simulink model "CSEI"  (Simulink 7.3)
settings: Solver=ode4  StartTime=0.0  StopTime=Inf  FixedStep=0.1  RelTol=1e-3
values from neighbouring files (symbols this model uses):
  Ke = 100*diag([1.28 1.05 1.28 1.05 2.14])    [data.m]    (also in parameeters.m = diag([1.28 1.05 1.28 1.05 2.14]))
  Te = [1     0       1       0       0 ... (first row only)    [data.m]    (also in parameeters.m = [1 0 1 0 0; 0 1 0 1 1; ly1 -lx1 -ly2 -lx2 lx3])
undefined symbols (not defined in the file or in its folder): D, M
libraries: marine_gnc x6, simulink x5, simulink_extras x4
(part 1 of 2)
settings Model: Creator=hakonnod  LastModifiedBy=mcl  BufferReuse=off
settings DataIOCC: LimitDataPoints=off  SaveOutput=off  SignalLogging=off  SaveTime=off
settings OptimizationCC: BlockReduction=off  BooleanDataType=off  ConditionallyExecuteInputs=off  OptimizeBlockIOStorage=off  BufferReuse=off  ExpressionFolding=off  EnableMemcpy=off  LocalBlockOutputs=off  InitFltsAndDblsToZero=on  SimCompilerOptimization=On
settings ModelReferenceCC: UpdateModelReferenceTargets=Force
settings SFSimCC: SimBuildMode=sf_nonincremental_build
settings RTWCC: SystemTargetFile=nidll.tlc  TemplateMakefile=nidll_vc.tmf  Description=NI Real-Time Target for Release 2007b or later  ProcessScript=nidll_make_rtw_hook
settings STFCustomTargetCC: MatFileLogging=on  SystemTargetFile=nidll.tlc

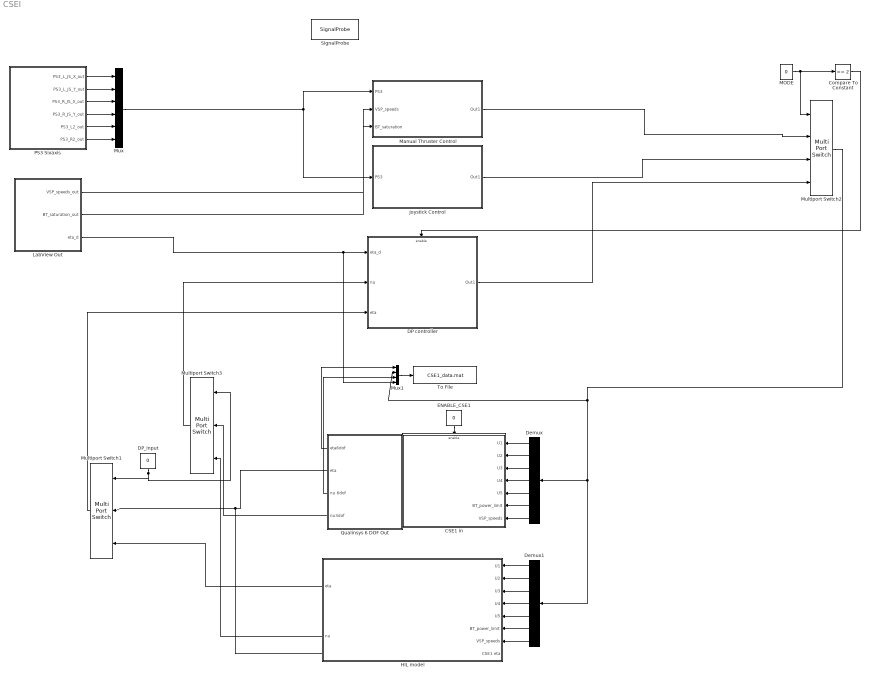
== system CSEI ==
  CSE1 in : Subsystem
  Compare To Constant : simulink/Logic and Bit Operations/Compare To Constant  SystemSampleTime=-1  relop===  const=2  LogicOutDataTypeMode=uint8
  DP controller : Subsystem
  DP_input : Constant  Value=0  OutDataType=fixdt(1, 16)  OutScaling=2^0
  Demux : Demux  Outputs=7
  Demux1 : Demux  Outputs=7
  ENABLE_CSE1 : Constant  Value=0  OutDataType=fixdt(1, 16)  OutScaling=2^0
  HIL model : Subsystem
  Joystick Control : Subsystem
  LabView Out : Subsystem
  MODE : Constant  Value=0  OutDataType=fixdt(1, 16)  OutScaling=2^0
  Manual Thruster Control : Subsystem
  Multiport Switch1 : MultiPortSwitch  Inputs=2  zeroidx=on  OutDataType=fixdt(1, 16)  OutScaling=2^0
  Multiport Switch2 : MultiPortSwitch  zeroidx=on  OutDataType=fixdt(1, 16)  OutScaling=2^0
  Multiport Switch3 : MultiPortSwitch  Inputs=2  zeroidx=on  OutDataType=fixdt(1, 16)  OutScaling=2^0
  Mux : Mux  Inputs=6
  Mux1 : Mux
  PS3 Sixaxis : Subsystem
  Qualinsys 6 DOF Out : Subsystem
  SignalProbe : S-Function  Description=Use this block with SIT.  FunctionName=SignalProbe  Parameters=1  EnableBusSupport=off
      settings: PreSaveFcn=NISIT_ModelVars;
      mask Description: The LabVIEW Simulation Interface Toolkit uses the SignalProbe block to probe the signals in the model. The SignalProbe block must be on the top level of the model hierarchy. You can have only one SignalProbe block per model file. Do not rename the SignalProbe block. Do not change the name of another model block to SignalProbe.
  To File : ToFile  Filename=CSE1_data.mat  MatrixName=cse1_data
  wires:
  PS3 Sixaxis/1(PS3_L_JS_X_out) -> Mux/1
  PS3 Sixaxis/2(PS3_L_JS_Y_out) -> Mux/2
  PS3 Sixaxis/3(PS3_R_JS_X_out) -> Mux/3
  PS3 Sixaxis/4(PS3_R_JS_Y_out) -> Mux/4
  PS3 Sixaxis/5(PS3_L2_out) -> Mux/5
  PS3 Sixaxis/6(PS3_R2_out) -> Mux/6
  Mux/1 -> Manual Thruster Control/1(PS3), Joystick Control/1(PS3)
  Manual Thruster Control/1(Out1) -> Multiport Switch2/2
  MODE/1 -> Multiport Switch2/1, Compare To Constant/1
  Multiport Switch2/1 -> Demux1/1, Demux/1, Mux1/2
  ENABLE_CSE1/1 -> CSE1 in/Enable
  DP controller/1(Out1) -> Multiport Switch2/4
  Compare To Constant/1 -> DP controller/Enable
  Joystick Control/1(Out1) -> Multiport Switch2/3
  Demux1/1 -> HIL model/1(U1)
  Demux1/2 -> HIL model/2(U2)
  Demux1/3 -> HIL model/3(U3)
  Demux1/4 -> HIL model/4(U4)
  Demux1/5 -> HIL model/5(U5)
  Demux1/6 -> HIL model/6(BT_power_limit)
  Demux1/7 -> HIL model/7(VSP_speeds)
  DP_input/1 -> Multiport Switch1/1, Multiport Switch3/1
  Qualinsys 6 DOF Out/2(eta) -> Multiport Switch1/2, HIL model/8(CSE1 eta)
  HIL model/1(eta) -> Multiport Switch1/3
  LabView Out/1(VSP_speeds_out) -> Manual Thruster Control/2(VSP_speeds)
  LabView Out/2(BT_saturation_out) -> Manual Thruster Control/3(BT_saturation)
  LabView Out/3(eta_d) -> DP controller/1(eta_d), Mux1/4
  HIL model/2(nu) -> Multiport Switch3/3
  Multiport Switch3/1 -> DP controller/2(nu)
  Mux1/1 -> To File/1
  Qualinsys 6 DOF Out/1(eta6dof) -> Mux1/1
  Demux/1 -> CSE1 in/1(U1)
  Demux/2 -> CSE1 in/2(U2)
  Demux/3 -> CSE1 in/3(U3)
  Demux/4 -> CSE1 in/4(U4)
  Demux/5 -> CSE1 in/5(U5)
  Demux/6 -> CSE1 in/6(BT_power_limit)
  Demux/7 -> CSE1 in/7(VSP_speeds)
  Qualinsys 6 DOF Out/4(nu3dof) -> Multiport Switch3/2
  Multiport Switch1/1 -> DP controller/3(eta)
  Qualinsys 6 DOF Out/3(nu 6dof) -> Mux1/3

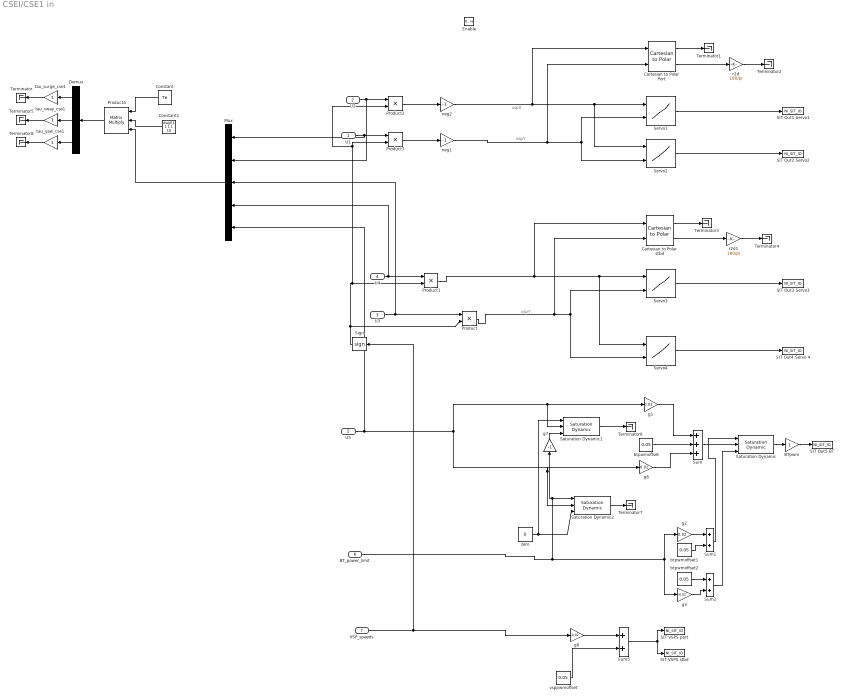
== system CSEI/CSE1 in ==
  note: vspX
  note: vspY
  note: vspY
  U1 : Inport  OutDataType=fixdt(1, 16)  OutScaling=2^0
  U2 : Inport  Port=2  OutDataType=fixdt(1, 16)  OutScaling=2^0
  U3 : Inport  Port=3  OutDataType=fixdt(1, 16)  OutScaling=2^0
  U4 : Inport  Port=4  OutDataType=fixdt(1, 16)  OutScaling=2^0
  U5 : Inport  Port=5  OutDataType=fixdt(1, 16)  OutScaling=2^0
  BT_power_limit : Inport  Port=6  OutDataType=fixdt(1, 16)  OutScaling=2^0
  VSP_speeds : Inport  Port=7  OutDataType=fixdt(1, 16)  OutScaling=2^0
  Enable : EnablePort
  BTpwm : Gain  ParameterDataType=fixdt(1, 16)  ParameterScaling=2^0  OutDataType=fixdt(1, 16)  OutScaling=2^0
  Cartesian to Polar Port : simulink_extras/Transformations/Cartesian to Polar  SystemSampleTime=-1
  Cartesian to Polar stbd : simulink_extras/Transformations/Cartesian to Polar  SystemSampleTime=-1
  Constant : Constant  Value=Te
  Constant1 : Constant  Value=diag([1 1 1 1 1])
  Demux : Demux  Outputs=3
  Mux : Mux  Inputs=5
  Product{,1..3} (4 alike) : Product  OutDataType=fixdt(1, 16)  OutScaling=2^0  RndMeth=Zero
  Product4 : Product  Inputs=3  Multiplication=Matrix(*)  RndMeth=Zero
  SIT Out1 Servo1 : S-Function  Priority=1  FunctionName=NI_SIT_IO  Parameters=width dtype portnum stime stype btype  EnableBusSupport=off  mask(SIT Outport){portnum=1, width=-1, stime=-1, dtype=auto, stype=auto, btype=0}
      mask prompts: portnum "Port number:"; width "Port dimensions (-1 for dynamically sized):"; stime "Sample time (-1 for inherited):"; dtype "Data type:"; stype "Signal type:"; btype "Block type:"
      mask help: Use this outport on any level of nested subsystems to allow the LabVIEW Simulation Interface Toolkit to map hardware to it.
      mask init:
      | NI_SIT_IO_init;
      settings: CopyFcn=NI_SIT_IO_callbacks(1);  DeleteFcn=NI_SIT_IO_callbacks(2);
      mask StyleString: edit,edit,edit,popup(auto|double|single|int8|uint8|int16|uint16|int32|uint32|boolean),popup(auto|real|complex),edit
      mask CallbackString: NI_SIT_IO_callbacks(3);|||NI_SIT_IO_callbacks(4);||
      mask TabNameString: Parameters,Parameters,Parameters,Parameters,Parameters,Parameters
      mask Display:
      | patch([-x x], [-y y], [.90980 .81960 .32156]);
      | plot([0 -x x 0], [rad -y y rad]);
      | fprintf('SIT%d', portnum);
  SIT Out2 Servo2 : S-Function  Priority=2  FunctionName=NI_SIT_IO  Parameters=width dtype portnum stime stype btype  EnableBusSupport=off  mask(SIT Outport){portnum=2, width=-1, stime=-1, dtype=auto, stype=auto, btype=0}
      mask prompts: portnum "Port number:"; width "Port dimensions (-1 for dynamically sized):"; stime "Sample time (-1 for inherited):"; dtype "Data type:"; stype "Signal type:"; btype "Block type:"
      mask help: Use this outport on any level of nested subsystems to allow the LabVIEW Simulation Interface Toolkit to map hardware to it.
      mask init:
      | NI_SIT_IO_init;
      settings: CopyFcn=NI_SIT_IO_callbacks(1);  DeleteFcn=NI_SIT_IO_callbacks(2);
      mask StyleString: edit,edit,edit,popup(auto|double|single|int8|uint8|int16|uint16|int32|uint32|boolean),popup(auto|real|complex),edit
      mask CallbackString: NI_SIT_IO_callbacks(3);|||NI_SIT_IO_callbacks(4);||
      mask TabNameString: Parameters,Parameters,Parameters,Parameters,Parameters,Parameters
      mask Display:
      | patch([-x x], [-y y], [.90980 .81960 .32156]);
      | plot([0 -x x 0], [rad -y y rad]);
      | fprintf('SIT%d', portnum);
  SIT Out3 Servo3 : S-Function  Priority=3  FunctionName=NI_SIT_IO  Parameters=width dtype portnum stime stype btype  EnableBusSupport=off  mask(SIT Outport){portnum=3, width=-1, stime=-1, dtype=auto, stype=auto, btype=0}
      mask prompts: portnum "Port number:"; width "Port dimensions (-1 for dynamically sized):"; stime "Sample time (-1 for inherited):"; dtype "Data type:"; stype "Signal type:"; btype "Block type:"
      mask help: Use this outport on any level of nested subsystems to allow the LabVIEW Simulation Interface Toolkit to map hardware to it.
      mask init:
      | NI_SIT_IO_init;
      settings: CopyFcn=NI_SIT_IO_callbacks(1);  DeleteFcn=NI_SIT_IO_callbacks(2);
      mask StyleString: edit,edit,edit,popup(auto|double|single|int8|uint8|int16|uint16|int32|uint32|boolean),popup(auto|real|complex),edit
      mask CallbackString: NI_SIT_IO_callbacks(3);|||NI_SIT_IO_callbacks(4);||
      mask TabNameString: Parameters,Parameters,Parameters,Parameters,Parameters,Parameters
      mask Display:
      | patch([-x x], [-y y], [.90980 .81960 .32156]);
      | plot([0 -x x 0], [rad -y y rad]);
      | fprintf('SIT%d', portnum);
  SIT Out4 Servo 4 : S-Function  Priority=4  FunctionName=NI_SIT_IO  Parameters=width dtype portnum stime stype btype  EnableBusSupport=off  mask(SIT Outport){portnum=4, width=-1, stime=-1, dtype=auto, stype=auto, btype=0}
      mask prompts: portnum "Port number:"; width "Port dimensions (-1 for dynamically sized):"; stime "Sample time (-1 for inherited):"; dtype "Data type:"; stype "Signal type:"; btype "Block type:"
      mask help: Use this outport on any level of nested subsystems to allow the LabVIEW Simulation Interface Toolkit to map hardware to it.
      mask init:
      | NI_SIT_IO_init;
      settings: CopyFcn=NI_SIT_IO_callbacks(1);  DeleteFcn=NI_SIT_IO_callbacks(2);
      mask StyleString: edit,edit,edit,popup(auto|double|single|int8|uint8|int16|uint16|int32|uint32|boolean),popup(auto|real|complex),edit
      mask CallbackString: NI_SIT_IO_callbacks(3);|||NI_SIT_IO_callbacks(4);||
      mask TabNameString: Parameters,Parameters,Parameters,Parameters,Parameters,Parameters
      mask Display:
      | patch([-x x], [-y y], [.90980 .81960 .32156]);
      | plot([0 -x x 0], [rad -y y rad]);
      | fprintf('SIT%d', portnum);
  SIT Out5 BT : S-Function  Priority=5  FunctionName=NI_SIT_IO  Parameters=width dtype portnum stime stype btype  EnableBusSupport=off  mask(SIT Outport){portnum=5, width=-1, stime=-1, dtype=auto, stype=auto, btype=0}
      mask prompts: portnum "Port number:"; width "Port dimensions (-1 for dynamically sized):"; stime "Sample time (-1 for inherited):"; dtype "Data type:"; stype "Signal type:"; btype "Block type:"
      mask help: Use this outport on any level of nested subsystems to allow the LabVIEW Simulation Interface Toolkit to map hardware to it.
      mask init:
      | NI_SIT_IO_init;
      settings: CopyFcn=NI_SIT_IO_callbacks(1);  DeleteFcn=NI_SIT_IO_callbacks(2);
      mask StyleString: edit,edit,edit,popup(auto|double|single|int8|uint8|int16|uint16|int32|uint32|boolean),popup(auto|real|complex),edit
      mask CallbackString: NI_SIT_IO_callbacks(3);|||NI_SIT_IO_callbacks(4);||
      mask TabNameString: Parameters,Parameters,Parameters,Parameters,Parameters,Parameters
      mask Display:
      | patch([-x x], [-y y], [.90980 .81960 .32156]);
      | plot([0 -x x 0], [rad -y y rad]);
      | fprintf('SIT%d', portnum);
  SIT VSPS port : S-Function  Priority=6  FunctionName=NI_SIT_IO  Parameters=width dtype portnum stime stype btype  EnableBusSupport=off  mask(SIT Outport){portnum=6, width=-1, stime=-1, dtype=auto, stype=auto, btype=0}
      mask prompts: portnum "Port number:"; width "Port dimensions (-1 for dynamically sized):"; stime "Sample time (-1 for inherited):"; dtype "Data type:"; stype "Signal type:"; btype "Block type:"
      mask help: Use this outport on any level of nested subsystems to allow the LabVIEW Simulation Interface Toolkit to map hardware to it.
      mask init:
      | NI_SIT_IO_init;
      settings: CopyFcn=NI_SIT_IO_callbacks(1);  DeleteFcn=NI_SIT_IO_callbacks(2);
      mask StyleString: edit,edit,edit,popup(auto|double|single|int8|uint8|int16|uint16|int32|uint32|boolean),popup(auto|real|complex),edit
      mask CallbackString: NI_SIT_IO_callbacks(3);|||NI_SIT_IO_callbacks(4);||
      mask TabNameString: Parameters,Parameters,Parameters,Parameters,Parameters,Parameters
      mask Display:
      | patch([-x x], [-y y], [.90980 .81960 .32156]);
      | plot([0 -x x 0], [rad -y y rad]);
      | fprintf('SIT%d', portnum);
  SIT VSPS stbd : S-Function  Priority=7  FunctionName=NI_SIT_IO  Parameters=width dtype portnum stime stype btype  EnableBusSupport=off  mask(SIT Outport){portnum=7, width=-1, stime=-1, dtype=auto, stype=auto, btype=0}
      mask prompts: portnum "Port number:"; width "Port dimensions (-1 for dynamically sized):"; stime "Sample time (-1 for inherited):"; dtype "Data type:"; stype "Signal type:"; btype "Block type:"
      mask help: Use this outport on any level of nested subsystems to allow the LabVIEW Simulation Interface Toolkit to map hardware to it.
      mask init:
      | NI_SIT_IO_init;
      settings: CopyFcn=NI_SIT_IO_callbacks(1);  DeleteFcn=NI_SIT_IO_callbacks(2);
      mask StyleString: edit,edit,edit,popup(auto|double|single|int8|uint8|int16|uint16|int32|uint32|boolean),popup(auto|real|complex),edit
      mask CallbackString: NI_SIT_IO_callbacks(3);|||NI_SIT_IO_callbacks(4);||
      mask TabNameString: Parameters,Parameters,Parameters,Parameters,Parameters,Parameters
      mask Display:
      | patch([-x x], [-y y], [.90980 .81960 .32156]);
      | plot([0 -x x 0], [rad -y y rad]);
      | fprintf('SIT%d', portnum);
  Saturation Dynamic : simulink/Discontinuities/Saturation Dynamic  SystemSampleTime=-1  OutMin=[]  OutMax=[]  OutDataTypeStr=Inherit: Same as second input  OutDataType=fixdt(1, 16)  OutScaling=2^-10  DoSatur=off
  Saturation Dynamic1 : simulink/Discontinuities/Saturation Dynamic  SystemSampleTime=-1  OutMin=[]  OutMax=[]  OutDataTypeStr=Inherit: Same as second input  OutDataType=fixdt(1, 16)  OutScaling=2^-10  DoSatur=off
  Saturation Dynamic2 : simulink/Discontinuities/Saturation Dynamic  SystemSampleTime=-1  OutMin=[]  OutMax=[]  OutDataTypeStr=Inherit: Same as second input  OutDataType=fixdt(1, 16)  OutScaling=2^-10  DoSatur=off
  Servo1 : Lookup2D  RowIndex=[-1,0,1]  ColumnIndex=[-1,0,1]  Table=reshape([0.06,0.0495363,0.043301,0.06,0.052446,0.043301,0.06,0.0541518,0.043301],3,3)  OutDataType=fixdt(1, 16)  OutScaling=2^0
  Servo2 : Lookup2D  RowIndex=[-1,0,1]  ColumnIndex=[-1,0,1]  Table=reshape([0.03860880,0.0386088,0.03860880,0.0459941,0.0477243,0.0500953,0.057,0.057,0.057],3,3)  OutDataType=fixdt(1, 16)  OutScaling=2^0
  Servo3 : Lookup2D  RowIndex=[-1,0,1]  ColumnIndex=[-1,0,1]  Table=reshape([0.0640809,0.0640809,0.0640809,0.0539629,0.0541315,0.0556492,0.0442664,0.0442664,0.0442664],3,3)  OutDataType=fixdt(1, 16)  OutScaling=2^0
  Servo4 : Lookup2D  RowIndex=[-1,0,1]  ColumnIndex=[-1,0,1]  Table=reshape([0.0602867,0.0470489,0.0403879,0.0602867,0.049747,0.0403879,0.0602867,0.0526138,0.0403879],3,3)  OutDataType=fixdt(1, 16)  OutScaling=2^0
  Sign : Signum
  Sum : Sum  Inputs=+++  OutDataType=fixdt(1, 16)  OutScaling=2^0
  Sum1 : Sum  OutDataType=fixdt(1, 16)  OutScaling=2^0
  Sum2 : Sum  OutDataType=fixdt(1, 16)  OutScaling=2^0
  Sum5 : Sum  OutDataType=fixdt(1, 16)  OutScaling=2^0
  Terminator{,1..8} (9 alike) : Terminator
  btpwmoffset : Constant  Value=0.05  OutDataType=fixdt(1, 16)  OutScaling=2^0
  btpwmoffset1 : Constant  Value=0.05  OutDataType=fixdt(1, 16)  OutScaling=2^0
  btpwmoffset2 : Constant  Value=0.05  OutDataType=fixdt(1, 16)  OutScaling=2^0
  g1 : Gain  Gain=0.02  ParameterDataType=fixdt(1, 16)  ParameterScaling=2^0  OutDataType=fixdt(1, 16)  OutScaling=2^0
  g2 : Gain  Gain=0.02  ParameterDataType=fixdt(1, 16)  ParameterScaling=2^0  OutDataType=fixdt(1, 16)  OutScaling=2^0
  g3 : Gain  Gain=-0.02  ParameterDataType=fixdt(1, 16)  ParameterScaling=2^0  OutDataType=fixdt(1, 16)  OutScaling=2^0
  g6 : Gain  Gain=0.02  ParameterDataType=fixdt(1, 16)  ParameterScaling=2^0  OutDataType=fixdt(1, 16)  OutScaling=2^0
  g7 : Gain  Gain=-1  ParameterDataType=fixdt(1, 16)  ParameterScaling=2^0  OutDataType=fixdt(1, 16)  OutScaling=2^0
  g8 : Gain  Gain=-0.02  ParameterDataType=fixdt(1, 16)  ParameterScaling=2^0  OutDataType=fixdt(1, 16)  OutScaling=2^0
  neg1 : Gain  Gain=-1  ParameterDataType=fixdt(1, 16)  ParameterScaling=2^0  OutDataType=fixdt(1, 16)  OutScaling=2^0
  neg2 : Gain  Gain=-1  ParameterDataType=fixdt(1, 16)  ParameterScaling=2^0  OutDataType=fixdt(1, 16)  OutScaling=2^0
  r2d : Gain  Gain=180/pi  ParameterDataType=fixdt(1, 16)  ParameterScaling=2^0  OutDataType=fixdt(1, 16)  OutScaling=2^0
  r2d1 : Gain  Gain=180/pi  ParameterDataType=fixdt(1, 16)  ParameterScaling=2^0  OutDataType=fixdt(1, 16)  OutScaling=2^0
  tau_surge_cse1 : Gain  ParameterDataType=fixdt(1, 16)  ParameterScaling=2^0  OutDataType=fixdt(1, 16)  OutScaling=2^0
  tau_sway_cse1 : Gain  ParameterDataType=fixdt(1, 16)  ParameterScaling=2^0  OutDataType=fixdt(1, 16)  OutScaling=2^0
  tau_yaw_cse1 : Gain  ParameterDataType=fixdt(1, 16)  ParameterScaling=2^0  OutDataType=fixdt(1, 16)  OutScaling=2^0
  vsppwmoffset : Constant  Value=0.05  OutDataType=fixdt(1, 16)  OutScaling=2^0
  zero : Constant  Value=0  OutDataType=fixdt(1, 16)  OutScaling=2^0
  wires:
  Servo1/1 -> SIT Out1 Servo1/1
  Servo2/1 -> SIT Out2 Servo2/1
  Cartesian to Polar Port/1 -> Terminator1/1
  Cartesian to Polar Port/2 -> r2d/1
  r2d/1 -> Terminator2/1
  neg2/1 -> Servo1/1, Servo2/1, Cartesian to Polar Port/1
  neg1/1 -> Servo1/2, Servo2/2, Cartesian to Polar Port/2
  Servo3/1 -> SIT Out3 Servo3/1
  Servo4/1 -> SIT Out4 Servo 4/1
  Cartesian to Polar stbd/1 -> Terminator3/1
  Cartesian to Polar stbd/2 -> r2d1/1
  r2d1/1 -> Terminator4/1
  BTpwm/1 -> SIT Out5 BT/1
  Sum/1 -> Saturation Dynamic/2
  Saturation Dynamic/1 -> BTpwm/1
  BT_power_limit/1 -> g2/1, g3/1, Saturation Dynamic2/1, g7/1
  btpwmoffset1/1 -> Sum1/2
  g2/1 -> Sum1/1
  Sum1/1 -> Saturation Dynamic/1
  g3/1 -> Sum2/2
  btpwmoffset2/1 -> Sum2/1
  Sum2/1 -> Saturation Dynamic/3
  Saturation Dynamic1/1 -> Terminator6/1
  Saturation Dynamic2/1 -> Terminator7/1
  zero/1 -> Saturation Dynamic2/3, Saturation Dynamic1/1
  g1/1 -> Sum/1
  btpwmoffset/1 -> Sum/2
  g6/1 -> Sum/3
  g7/1 -> Saturation Dynamic1/3
  U5/1 -> Saturation Dynamic1/2, g1/1, Saturation Dynamic2/2, g6/1, Mux/5
  vsppwmoffset/1 -> Sum5/2
  Sum5/1 -> SIT VSPS port/1, SIT VSPS stbd/1
  g8/1 -> Sum5/1
  VSP_speeds/1 -> g8/1, Sign/1
  U3/1 -> Product/1, Mux/3
  Product/1 -> Servo3/2, Servo4/2, Cartesian to Polar stbd/2
  Sign/1 -> Product/2, Product1/2, Product3/2, Product2/2
  U4/1 -> Product1/1, Mux/4
  Product1/1 -> Servo3/1, Servo4/1, Cartesian to Polar stbd/1
  U2/1 -> Product2/1, Mux/2
  U1/1 -> Product3/1, Mux/1
  Product2/1 -> neg2/1
  Product3/1 -> neg1/1
  Constant1/1 -> Product4/2
  Constant/1 -> Product4/1
  Demux/1 -> tau_surge_cse1/1
  Demux/2 -> tau_sway_cse1/1
  Demux/3 -> tau_yaw_cse1/1
  Product4/1 -> Demux/1
  tau_surge_cse1/1 -> Terminator/1
  tau_sway_cse1/1 -> Terminator5/1
  tau_yaw_cse1/1 -> Terminator8/1
  Mux/1 -> Product4/3

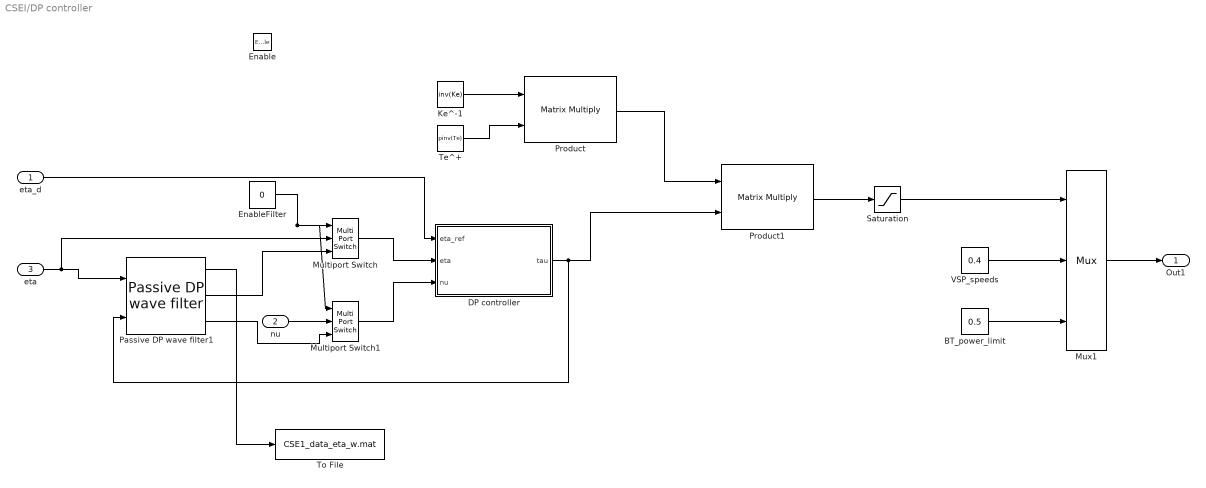
== system CSEI/DP controller ==
  eta_d : Inport  OutDataType=fixdt(1, 16)  OutScaling=2^0
  nu : Inport  Port=2  OutDataType=fixdt(1, 16)  OutScaling=2^0
  eta : Inport  Port=3  OutDataType=fixdt(1, 16)  OutScaling=2^0
  Enable : EnablePort  StatesWhenEnabling=reset
  BT_power_limit : Constant  Value=0.5  OutDataType=fixdt(1, 16)  OutScaling=2^0
  DP controller : Subsystem  mask(Nonlinear DP Controller){Kp=(0.1)^2*[25.8000 0  0;  0  33.8000  1.0115;  0  1.0115  2.7600 ], Kd=2*0.8*0.1*[25.8000 0  0;  0  33.8000  1.0115;  0  1.0115  2.7600 ], Ki=(0.1^3/10)*[25.8000 0  0;  0  33.8000  1.0115;  0  1.0115  2.7600 ]}
      mask prompts: Kp "Proportional Gain Matrix: Kp"; Kd "Derivative Gain Matrix: Kd"; Ki "Integral Gain Matrix: Ki"
      mask help: Nonlinear PID controller for Set-Point Reulation in Surge, Sway and Yaw
      mask Help:
      | The nonlinear  PID controller uses the rotation matrix in yaw for proper scaling of the surge, sway and yaw gains as a function of the yaw angle.
      | INPUTS: (1) eta_ref, (2) eta, (3) nu. OUPUTS: (1) tau.
      mask Display: disp('Nonlinear PID\n set-point controller')
  EnableFilter : Constant  Value=0  OutDataType=fixdt(1, 16)  OutScaling=2^0
  Ke^-1 : Constant  Value=inv(Ke)  OutDataType=fixdt(1, 16)  OutScaling=2^0
  Multiport Switch : MultiPortSwitch  Inputs=2  zeroidx=on  OutDataType=fixdt(1, 16)  OutScaling=2^0
  Multiport Switch1 : MultiPortSwitch  Inputs=2  zeroidx=on  OutDataType=fixdt(1, 16)  OutScaling=2^0
  Mux1 : Mux  Inputs=3
  Passive DP wave filter1 : marine_gnc/Navigation/Observers/Passive DP wave filter  SystemSampleTime=-1  lambda=0.1*diag([1 1 1])  w_o=diag([0.8 0.8 0.8])  K4=0.1*diag([1 1 0.1])  K3=0.1*diag([1 1 0.1])  w_c=1.3*diag([0.8 0.8 0.8])  T_b=diag([100 100 100])  M="[ 25.8000   0    0;   0   33.8000   1.0115; 0   1.0115    2.7600 ]"  D="[2 0  0;  0 7 0.1; 0 0.1 0.5]"
  Product : Product  Multiplication=Matrix(*)  OutDataType=fixdt(1, 16)  OutScaling=2^0  RndMeth=Zero
  Product1 : Product  Multiplication=Matrix(*)  OutDataType=fixdt(1, 16)  OutScaling=2^0  RndMeth=Zero
  Saturation : Saturate  UpperLimit=1.0  LowerLimit=-1.0  OutDataType=fixdt(1, 16)  OutScaling=2^0
  Te^+ : Constant  Value=pinv(Te)  OutDataType=fixdt(1, 16)  OutScaling=2^0
  To File : ToFile  Filename=CSE1_data_eta_w.mat  MatrixName=cse1_data
  VSP_speeds : Constant  Value=0.4  OutDataType=fixdt(1, 16)  OutScaling=2^0
  Out1 : Outport  OutDataType=fixdt(1, 16)  OutScaling=2^0
  wires:
  Product/1 -> Product1/1
  DP controller/1(tau) -> Product1/2, Passive DP wave filter1/2
  Ke^-1/1 -> Product/1
  Te^+/1 -> Product/2
  Mux1/1 -> Out1/1
  VSP_speeds/1 -> Mux1/2
  BT_power_limit/1 -> Mux1/3
  eta_d/1 -> DP controller/1(eta_ref)
  eta/1 -> Passive DP wave filter1/1, Multiport Switch/2
  nu/1 -> Multiport Switch1/2
  Multiport Switch/1 -> DP controller/2(eta)
  Multiport Switch1/1 -> DP controller/3(nu)
  Passive DP wave filter1/2 -> Multiport Switch/3
  Passive DP wave filter1/3 -> Multiport Switch1/3
  EnableFilter/1 -> Multiport Switch/1, Multiport Switch1/1
  Product1/1 -> Saturation/1
  Saturation/1 -> Mux1/1
  Passive DP wave filter1/1 -> To File/1

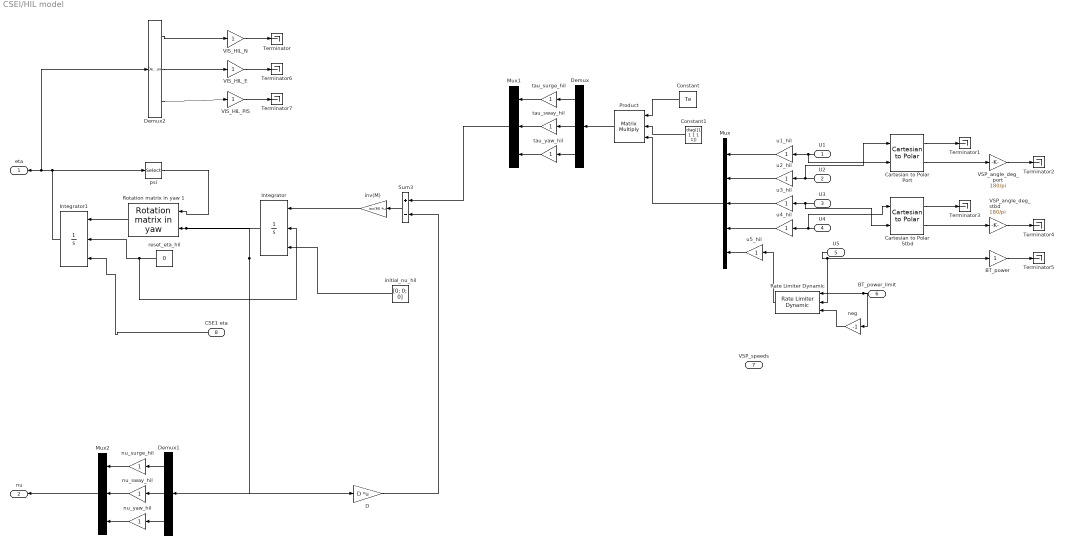
== system CSEI/HIL model ==
  U1 : Inport  OutDataType=fixdt(1, 16)  OutScaling=2^0
  U2 : Inport  Port=2  OutDataType=fixdt(1, 16)  OutScaling=2^0
  U3 : Inport  Port=3  OutDataType=fixdt(1, 16)  OutScaling=2^0
  U4 : Inport  Port=4  OutDataType=fixdt(1, 16)  OutScaling=2^0
  U5 : Inport  Port=5  OutDataType=fixdt(1, 16)  OutScaling=2^0
  BT_power_limit : Inport  Port=6  OutDataType=fixdt(1, 16)  OutScaling=2^0
  VSP_speeds : Inport  Port=7  OutDataType=fixdt(1, 16)  OutScaling=2^0
  CSE1 eta : Inport  Port=8  OutDataType=fixdt(1, 16)  OutScaling=2^0
  BT_power : Gain  ParameterDataType=fixdt(1, 16)  ParameterScaling=2^0  OutDataType=fixdt(1, 16)  OutScaling=2^0
  Cartesian to Polar Port : simulink_extras/Transformations/Cartesian to Polar  SystemSampleTime=-1
  Cartesian to Polar Stbd : simulink_extras/Transformations/Cartesian to Polar  SystemSampleTime=-1
  Constant : Constant  Value=Te
  Constant1 : Constant  Value=diag([1 1 1 1 1])
  D : Gain  Gain=D  Multiplication=Matrix(K*u)  ParameterDataType=sfix(16)  ParameterScaling=2^0  OutDataType=sfix(16)  OutScaling=2^0  SaturateOnIntegerOverflow=on  OutDataTypeStr=Inherit: Same as input  ParamDataTypeStr=Inherit: Same as input
  Demux : Demux  Outputs=3
  Demux1 : Demux  Outputs=3
  Demux2 : Demux  Outputs=3
  Integrator : Integrator  ExternalReset=level  InitialConditionSource=external
  Integrator1 : Integrator  ExternalReset=level  InitialConditionSource=external
  Mux : Mux  Inputs=5
  Mux1 : Mux  Inputs=3
  Mux2 : Mux  Inputs=3
  Product : Product  Inputs=3  Multiplication=Matrix(*)  RndMeth=Zero
  Rate Limiter Dynamic : simulink/Discontinuities/Rate Limiter Dynamic  SystemSampleTime=-1
  Rotation matrix in yaw 1 : marine_gnc/Models/ Kinematics/Rotation matrix in yaw   SystemSampleTime=-1
  Sum3 : Sum  Inputs=+-  OutDataType=sfix(16)  OutScaling=2^0  SaturateOnIntegerOverflow=on  InputSameDT=on  OutDataTypeStr=Inherit: Same as first input
  Terminator{,1..7} (8 alike) : Terminator
  VIS_HIL_E : Gain  ParameterDataType=fixdt(1, 16)  ParameterScaling=2^0  OutDataType=fixdt(1, 16)  OutScaling=2^0
  VIS_HIL_N : Gain  ParameterDataType=fixdt(1, 16)  ParameterScaling=2^0  OutDataType=fixdt(1, 16)  OutScaling=2^0
  VIS_HIL_PIS : Gain  ParameterDataType=fixdt(1, 16)  ParameterScaling=2^0  OutDataType=fixdt(1, 16)  OutScaling=2^0
  VSP_angle_deg_port : Gain  Gain=180/pi  ParameterDataType=fixdt(1, 16)  ParameterScaling=2^0  OutDataType=fixdt(1, 16)  OutScaling=2^0
  VSP_angle_deg_stbd : Gain  Gain=180/pi  ParameterDataType=fixdt(1, 16)  ParameterScaling=2^0  OutDataType=fixdt(1, 16)  OutScaling=2^0
  initial_nu_hil : Constant  Value=[0; 0; 0]  OutDataType=fixdt(1, 16)  OutScaling=2^0
  inv(M) : Gain  Gain=inv(M)  Multiplication=Matrix(K*u)  ParameterDataType=sfix(16)  ParameterScaling=2^0  OutDataType=sfix(16)  OutScaling=2^0  SaturateOnIntegerOverflow=on  OutDataTypeStr=Inherit: Same as input  ParamDataTypeStr=Inherit: Same as input
  neg : Gain  Gain=-1  ParameterDataType=fixdt(1, 16)  ParameterScaling=2^0  OutDataType=fixdt(1, 16)  OutScaling=2^0
  nu_surge_hil : Gain  ParameterDataType=fixdt(1, 16)  ParameterScaling=2^0  OutDataType=fixdt(1, 16)  OutScaling=2^0
  nu_sway_hil : Gain  ParameterDataType=fixdt(1, 16)  ParameterScaling=2^0  OutDataType=fixdt(1, 16)  OutScaling=2^0
  nu_yaw_hil : Gain  ParameterDataType=fixdt(1, 16)  ParameterScaling=2^0  OutDataType=fixdt(1, 16)  OutScaling=2^0
  psi : Selector  InputPortWidth=3  IndexOptions=Index vector (dialog)  Indices=[3]  OutputSizes=1
  reset_eta_hil : Constant  Value=0  OutDataType=fixdt(1, 16)  OutScaling=2^0
  tau_surge_hil : Gain  ParameterDataType=fixdt(1, 16)  ParameterScaling=2^0  OutDataType=fixdt(1, 16)  OutScaling=2^0
  tau_sway_hil : Gain  ParameterDataType=fixdt(1, 16)  ParameterScaling=2^0  OutDataType=fixdt(1, 16)  OutScaling=2^0
  tau_yaw_hil : Gain  ParameterDataType=fixdt(1, 16)  ParameterScaling=2^0  OutDataType=fixdt(1, 16)  OutScaling=2^0
  u1_hil : Gain  ParameterDataType=fixdt(1, 16)  ParameterScaling=2^0  OutDataType=fixdt(1, 16)  OutScaling=2^0
  u2_hil : Gain  ParameterDataType=fixdt(1, 16)  ParameterScaling=2^0  OutDataType=fixdt(1, 16)  OutScaling=2^0
  u3_hil : Gain  ParameterDataType=fixdt(1, 16)  ParameterScaling=2^0  OutDataType=fixdt(1, 16)  OutScaling=2^0
  u4_hil : Gain  ParameterDataType=fixdt(1, 16)  ParameterScaling=2^0  OutDataType=fixdt(1, 16)  OutScaling=2^0
  u5_hil : Gain  ParameterDataType=fixdt(1, 16)  ParameterScaling=2^0  OutDataType=fixdt(1, 16)  OutScaling=2^0
  eta : Outport  OutDataType=sfix(16)  OutScaling=2^0
  nu : Outport  Port=2  OutDataType=sfix(16)  OutScaling=2^0
  wires:
  Integrator/1 -> Rotation matrix in yaw 1/2, D/1, Demux1/1
  D/1 -> Sum3/2
  Sum3/1 -> inv(M)/1
  Rotation matrix in yaw 1/1 -> Integrator1/1
  psi/1 -> Rotation matrix in yaw 1/1
  Constant1/1 -> Product/2
  Mux/1 -> Product/3
  Constant/1 -> Product/1
  inv(M)/1 -> Integrator/1
  initial_nu_hil/1 -> Integrator/3
  U1/1 -> u1_hil/1, Cartesian to Polar Port/2
  U2/1 -> u2_hil/1, Cartesian to Polar Port/1
  U3/1 -> u3_hil/1, Cartesian to Polar Stbd/2
  U4/1 -> u4_hil/1, Cartesian to Polar Stbd/1
  U5/1 -> BT_power/1, Rate Limiter Dynamic/2
  Demux/1 -> tau_surge_hil/1
  tau_surge_hil/1 -> Mux1/1
  Demux/2 -> tau_sway_hil/1
  tau_sway_hil/1 -> Mux1/2
  Demux/3 -> tau_yaw_hil/1
  tau_yaw_hil/1 -> Mux1/3
  Product/1 -> Demux/1
  u1_hil/1 -> Mux/1
  u2_hil/1 -> Mux/2
  u3_hil/1 -> Mux/3
  u4_hil/1 -> Mux/4
  u5_hil/1 -> Mux/5
  Demux1/1 -> nu_surge_hil/1
  nu_surge_hil/1 -> Mux2/1
  Demux1/2 -> nu_sway_hil/1
  nu_sway_hil/1 -> Mux2/2
  Demux1/3 -> nu_yaw_hil/1
  nu_yaw_hil/1 -> Mux2/3
  Mux2/1 -> nu/1
  Mux1/1 -> Sum3/1
  Cartesian to Polar Port/1 -> Terminator1/1
  Cartesian to Polar Port/2 -> VSP_angle_deg_port/1
  VSP_angle_deg_port/1 -> Terminator2/1
  Cartesian to Polar Stbd/1 -> Terminator3/1
  Cartesian to Polar Stbd/2 -> VSP_angle_deg_stbd/1
  VSP_angle_deg_stbd/1 -> Terminator4/1
  BT_power/1 -> Terminator5/1
  Integrator1/1 -> psi/1, eta/1, Demux2/1
  reset_eta_hil/1 -> Integrator1/2, Integrator/2
  CSE1 eta/1 -> Integrator1/3
  VIS_HIL_N/1 -> Terminator/1
  Demux2/1 -> VIS_HIL_N/1
  VIS_HIL_E/1 -> Terminator6/1
  VIS_HIL_PIS/1 -> Terminator7/1
  Demux2/2 -> VIS_HIL_E/1
  Demux2/3 -> VIS_HIL_PIS/1
  Rate Limiter Dynamic/1 -> u5_hil/1
  BT_power_limit/1 -> Rate Limiter Dynamic/1, neg/1
  neg/1 -> Rate Limiter Dynamic/3

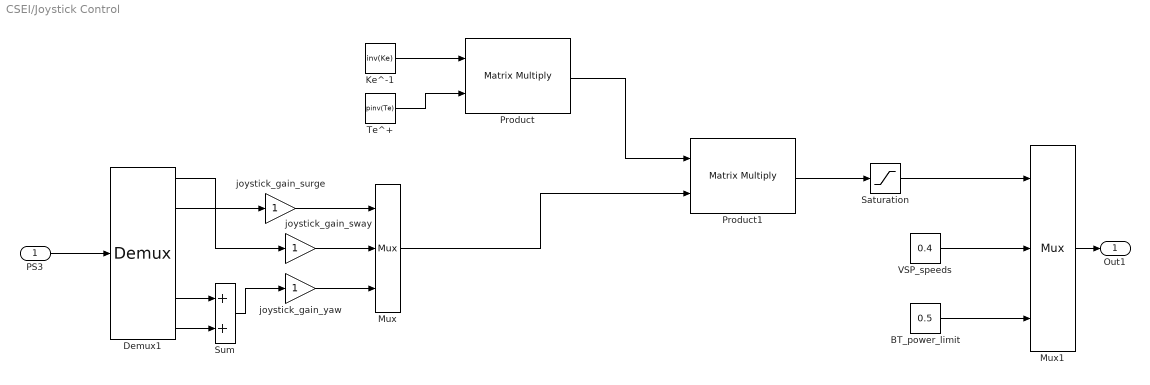
== system CSEI/Joystick Control ==
  PS3 : Inport  OutDataType=fixdt(1, 16)  OutScaling=2^0
  BT_power_limit : Constant  Value=0.5  OutDataType=fixdt(1, 16)  OutScaling=2^0
  Demux1 : Demux  Outputs=6
  Ke^-1 : Constant  Value=inv(Ke)  OutDataType=fixdt(1, 16)  OutScaling=2^0
  Mux : Mux  Inputs=3
  Mux1 : Mux  Inputs=3
  Product : Product  Multiplication=Matrix(*)  OutDataType=fixdt(1, 16)  OutScaling=2^0  RndMeth=Zero
  Product1 : Product  Multiplication=Matrix(*)  OutDataType=fixdt(1, 16)  OutScaling=2^0  RndMeth=Zero
  Saturation : Saturate  UpperLimit=1.0  LowerLimit=-1.0  OutDataType=fixdt(1, 16)  OutScaling=2^0
  Sum : Sum  OutDataType=fixdt(1, 16)  OutScaling=2^0
  Te^+ : Constant  Value=pinv(Te)  OutDataType=fixdt(1, 16)  OutScaling=2^0
  VSP_speeds : Constant  Value=0.4  OutDataType=fixdt(1, 16)  OutScaling=2^0
  joystick_gain_surge : Gain  ParameterDataType=fixdt(1, 16)  ParameterScaling=2^0  OutDataType=fixdt(1, 16)  OutScaling=2^0
  joystick_gain_sway : Gain  ParameterDataType=fixdt(1, 16)  ParameterScaling=2^0  OutDataType=fixdt(1, 16)  OutScaling=2^0
  joystick_gain_yaw : Gain  ParameterDataType=fixdt(1, 16)  ParameterScaling=2^0  OutDataType=fixdt(1, 16)  OutScaling=2^0
  Out1 : Outport  OutDataType=fixdt(1, 16)  OutScaling=2^0
  wires:
  PS3/1 -> Demux1/1
  Demux1/1 -> joystick_gain_sway/1
  Demux1/2 -> joystick_gain_surge/1
  Demux1/5 -> Sum/1
  Demux1/6 -> Sum/2
  Sum/1 -> joystick_gain_yaw/1
  Ke^-1/1 -> Product/1
  Te^+/1 -> Product/2
  Product/1 -> Product1/1
  joystick_gain_surge/1 -> Mux/1
  joystick_gain_sway/1 -> Mux/2
  joystick_gain_yaw/1 -> Mux/3
  Mux/1 -> Product1/2
  Mux1/1 -> Out1/1
  VSP_speeds/1 -> Mux1/2
  BT_power_limit/1 -> Mux1/3
  Product1/1 -> Saturation/1
  Saturation/1 -> Mux1/1

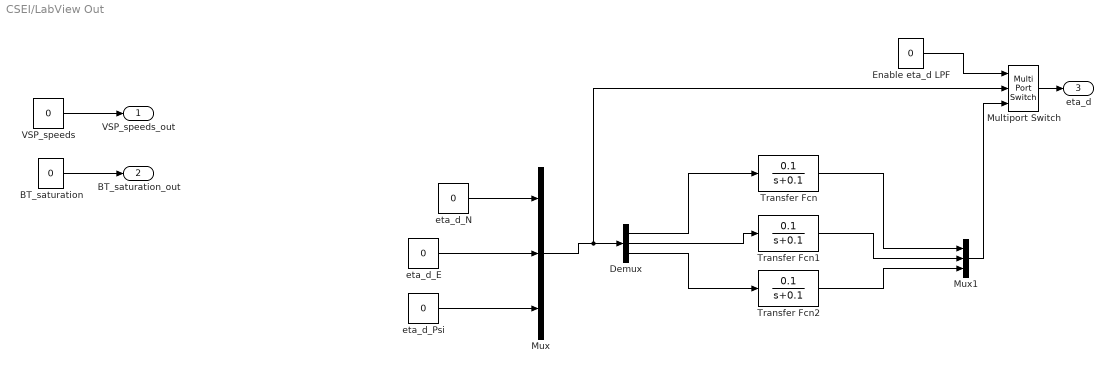
== system CSEI/LabView Out ==
  BT_saturation : Constant  Value=0  OutDataType=fixdt(1, 16)  OutScaling=2^0
  Demux : Demux  Outputs=3
  Enable eta_d LPF : Constant  Value=0  OutDataType=fixdt(1, 16)  OutScaling=2^0
  Multiport Switch : MultiPortSwitch  Inputs=2  zeroidx=on  OutDataType=fixdt(1, 16)  OutScaling=2^0
  Mux : Mux  Inputs=3
  Mux1 : Mux  Inputs=3
  Transfer Fcn : TransferFcn  Numerator=[0.1]  Denominator=[1 0.1]
  Transfer Fcn1 : TransferFcn  Numerator=[0.1]  Denominator=[1 0.1]
  Transfer Fcn2 : TransferFcn  Numerator=[0.1]  Denominator=[1 0.1]
  VSP_speeds : Constant  Value=0  OutDataType=fixdt(1, 16)  OutScaling=2^0
  eta_d_E : Constant  Value=0  OutDataType=fixdt(1, 16)  OutScaling=2^0
  eta_d_N : Constant  Value=0  OutDataType=fixdt(1, 16)  OutScaling=2^0
  eta_d_Psi : Constant  Value=0  OutDataType=fixdt(1, 16)  OutScaling=2^0
  VSP_speeds_out : Outport  OutDataType=fixdt(1, 16)  OutScaling=2^0
  BT_saturation_out : Outport  Port=2  OutDataType=fixdt(1, 16)  OutScaling=2^0
  eta_d : Outport  Port=3  OutDataType=fixdt(1, 16)  OutScaling=2^0
  wires:
  VSP_speeds/1 -> VSP_speeds_out/1
  BT_saturation/1 -> BT_saturation_out/1
  eta_d_N/1 -> Mux/1
  eta_d_E/1 -> Mux/2
  eta_d_Psi/1 -> Mux/3
  Demux/1 -> Transfer Fcn/1
  Transfer Fcn/1 -> Mux1/1
  Demux/2 -> Transfer Fcn1/1
  Transfer Fcn1/1 -> Mux1/2
  Demux/3 -> Transfer Fcn2/1
  Transfer Fcn2/1 -> Mux1/3
  Mux/1 -> Demux/1, Multiport Switch/2
  Mux1/1 -> Multiport Switch/3
  Enable eta_d LPF/1 -> Multiport Switch/1
  Multiport Switch/1 -> eta_d/1

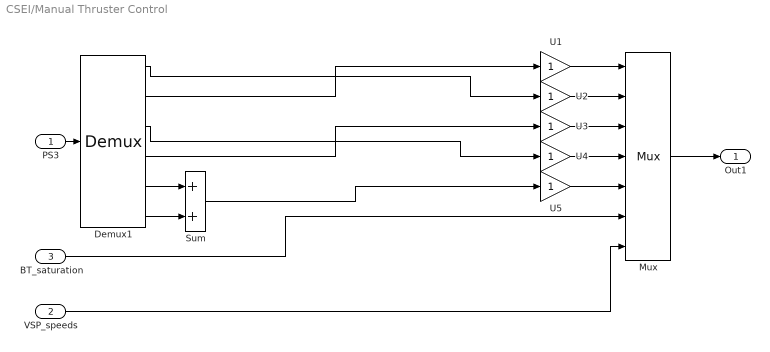
== system CSEI/Manual Thruster Control ==
  PS3 : Inport  OutDataType=fixdt(1, 16)  OutScaling=2^0
  VSP_speeds : Inport  Port=2  OutDataType=fixdt(1, 16)  OutScaling=2^0
  BT_saturation : Inport  Port=3  OutDataType=fixdt(1, 16)  OutScaling=2^0
  Demux1 : Demux  Outputs=6
  Mux : Mux  Inputs=7
  Sum : Sum  OutDataType=fixdt(1, 16)  OutScaling=2^0
  U{1..5} (5 alike) : Gain  ParameterDataType=fixdt(1, 16)  ParameterScaling=2^0  OutDataType=fixdt(1, 16)  OutScaling=2^0
  Out1 : Outport  OutDataType=fixdt(1, 16)  OutScaling=2^0
  wires:
  Mux/1 -> Out1/1
  PS3/1 -> Demux1/1
  Demux1/5 -> Sum/1
  Demux1/6 -> Sum/2
  Sum/1 -> U5/1
  BT_saturation/1 -> Mux/6
  VSP_speeds/1 -> Mux/7
  U1/1 -> Mux/1
  U2/1 -> Mux/2
  U3/1 -> Mux/3
  U4/1 -> Mux/4
  U5/1 -> Mux/5
  Demux1/2 -> U1/1
  Demux1/1 -> U2/1
  Demux1/4 -> U3/1
  Demux1/3 -> U4/1

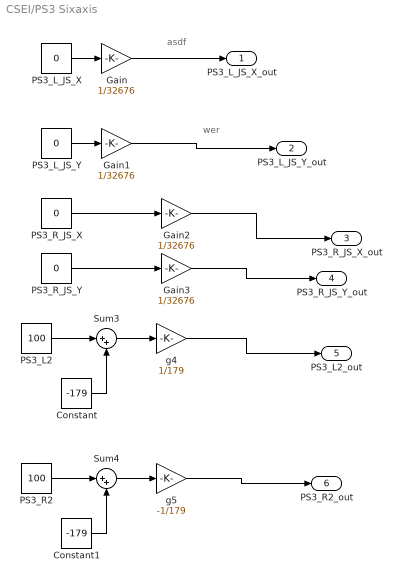
== system CSEI/PS3 Sixaxis ==
  note: asdf
  note: wer
  Constant : Constant  Value=-179  OutDataType=fixdt(1, 16)  OutScaling=2^0
  Constant1 : Constant  Value=-179  OutDataType=fixdt(1, 16)  OutScaling=2^0
  Gain{,1..3} (4 alike) : Gain  Gain=1/32676  ParameterDataType=fixdt(1, 16)  ParameterScaling=2^0  OutDataType=fixdt(1, 16)  OutScaling=2^0
  PS3_L2 : Constant  Value=100  OutDataType=fixdt(1, 16)  OutScaling=2^0
  PS3_L_JS_X : Constant  Value=0  OutDataType=fixdt(1, 16)  OutScaling=2^0
  PS3_L_JS_Y : Constant  Value=0  OutDataType=fixdt(1, 16)  OutScaling=2^0
  PS3_R2 : Constant  Value=100  OutDataType=fixdt(1, 16)  OutScaling=2^0
  PS3_R_JS_X : Constant  Value=0  OutDataType=fixdt(1, 16)  OutScaling=2^0
  PS3_R_JS_Y : Constant  Value=0  OutDataType=fixdt(1, 16)  OutScaling=2^0
  Sum3 : Sum  Inputs=|++  OutDataType=fixdt(1, 16)  OutScaling=2^0
  Sum4 : Sum  Inputs=|++  OutDataType=fixdt(1, 16)  OutScaling=2^0
  g4 : Gain  Gain=1/179  ParameterDataType=fixdt(1, 16)  ParameterScaling=2^0  OutDataType=fixdt(1, 16)  OutScaling=2^0
  g5 : Gain  Gain=-1/179  ParameterDataType=fixdt(1, 16)  ParameterScaling=2^0  OutDataType=fixdt(1, 16)  OutScaling=2^0
  PS3_L_JS_X_out : Outport  OutDataType=fixdt(1, 16)  OutScaling=2^0
  PS3_L_JS_Y_out : Outport  Port=2  OutDataType=fixdt(1, 16)  OutScaling=2^0
  PS3_R_JS_X_out : Outport  Port=3  OutDataType=fixdt(1, 16)  OutScaling=2^0
  PS3_R_JS_Y_out : Outport  Port=4  OutDataType=fixdt(1, 16)  OutScaling=2^0
  PS3_L2_out : Outport  Port=5  OutDataType=fixdt(1, 16)  OutScaling=2^0
  PS3_R2_out : Outport  Port=6  OutDataType=fixdt(1, 16)  OutScaling=2^0
  wires:
  PS3_L_JS_Y/1 -> Gain1/1
  PS3_L_JS_X/1 -> Gain/1
  PS3_R_JS_Y/1 -> Gain3/1
  PS3_R_JS_X/1 -> Gain2/1
  PS3_L2/1 -> Sum3/1
  Constant/1 -> Sum3/2
  Sum3/1 -> g4/1
  PS3_R2/1 -> Sum4/1
  Constant1/1 -> Sum4/2
  Sum4/1 -> g5/1
  Gain/1 -> PS3_L_JS_X_out/1
  Gain1/1 -> PS3_L_JS_Y_out/1
  Gain2/1 -> PS3_R_JS_X_out/1
  Gain3/1 -> PS3_R_JS_Y_out/1
  g4/1 -> PS3_L2_out/1
  g5/1 -> PS3_R2_out/1
